simulink model "ng_pv_dynamic_dbus_p_1_sm_ng"  (Simulink 8.8)
settings: Solver=ode4  StartTime=0.0  StopTime=inf  FixedStep=0.000125  RelTol=1e-3  EnableMultiTasking=on
PreLoadFcn:
  | Ts=125e-6;Core_Num = 0; np=1; nq=1; Vmin=.9;
PostLoadFcn:
  | Ts=125e-6;Core_Num = 0; np=1; nq=1; Vmin=.9;
InitFcn:
  | Ts=125e-6;Core_Num = 0; np=1; nq=1; Vmin=.9;
undefined symbols (not defined in the file or in its folder): another_event_name, DiscIntNeverNeededParam, I, j, Left, my_event_name, Right, type, V, X
libraries: powerlib x316, simulink_extras x78, powerlib_meascontrol x47, ssn_lib x9, opal_lib x5, powerlib_extras x3, simulink x3, artemis x1, rtio_opalrt_ml605ex1 x1, rtlab x1, rtio_spectracom x1
(part 1 of 11)
settings Model: ARTEMISmethode_block_infos=$$__separator__$$ng_pv_dynamic_dbus_p_1_sm_ng/ARTEMIS Guide1$$__separator__$$  Creator=DETLDAQ  LastModifiedBy=DETLDAQ
settings OptimizationCC: BlockReduction=off  BooleanDataType=off  OptimizeBlockIOStorage=off  BufferReuse=off  GlobalBufferReuse=off  ExpressionFolding=off  LocalBlockOutputs=off
settings DebuggingCC: SaveWithParameterizedLinksMsg=none  SignalResolutionControl=TryResolveAllWithWarning  MultiTaskDSMMsg=warning  MultiTaskCondExecSysMsg=none  FcnCallInpInsideContextMsg=error
settings HardwareCC: TargetBitPerPointer=64  TargetBitPerSizeT=64  TargetBitPerPtrDiffT=64  TargetLongLongMode=on  TargetIntDivRoundTo=Zero  TargetEndianess=LittleEndian  TargetWordSize=64  TargetHWDeviceType=MATLAB Host  ProdEqTarget=off
settings RTWCC: GenCodeOnly=on
settings GRTTargetCC: CombineOutputUpdateFcns=on  GRTInterface=off

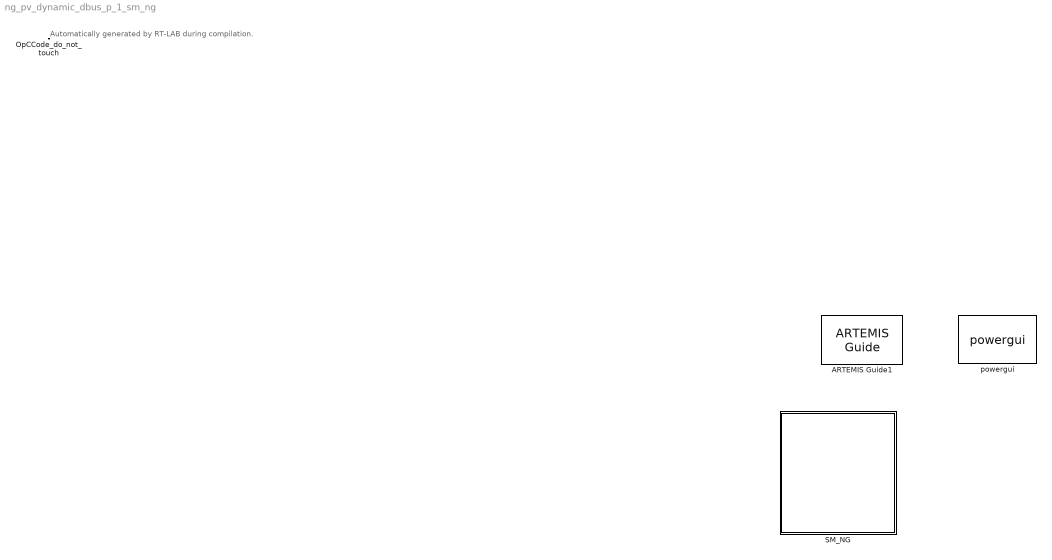
== system ng_pv_dynamic_dbus_p_1_sm_ng ==
  note: Automatically generated by RT-LAB during compilation.
  ARTEMIS Guide1 : artemis/ARTEMIS/ARTEMIS Guide  Tag=FTSSmethode_opal_4hx0r99  Description=5.0_z1  lock=on  Ts=Ts  opt=art5  dyna=off  nb_perm=4  RT_fullcomp=off  ssn=on  ssn_itvc=off  ssn_ivic=off  ssn_ext=off  ssn_solver=Backward Euler  ssn_impulse=off  ssn_quasimpulse=off  ssn_impulse_loop=5  paraExtinctionThy=off  Thy_Impulse=off  dtc=Off  dtc_opt=normal  ao=on  simtype=off  ct_mac=off  lin_mov=off  lsp=[0.001 2]  spike_skip=Disabled  dtc_extra=1  dtc_sws=normal  dtc_pied=0.5  SPSRulesBlock=SPSRules  tre=off  ctmm=off  LF=on  dpl_type=ARTEMiS DPL  rlc_type=off  custom_type=off  para=on  ssn_ImpulseLoopBlockedStateUpdate=5  ssn_mov_iter_number=5  ssn_switch_iter_number=5  ssn_nib_type_verify=on  ssn_use_lu=on  ssn_use_ldlt=off
  OpCCode_do_not_touch : opal_lib/Communication/OpCCode  SystemSampleTime=-1
  SM_NG : Subsystem
  powergui : powerlib/powergui  SimulationMode=Discrete  SolverType=Backward Euler  SampleTime=0.000125  frequency=60  SPID=off  DisableSnubberDevices=off  DisableRonSwitches=off  DisableVfSwitches=off  SwTol=0  DisplayEquations=off  Interpol=off  ExternalGateDelay=off  methode=off  Ts=100  FunctionMessages=off  echomessages=off  HookPort=off  EnableUseOfTLC=off  x0status=blocks  frequencyindice=0  Pbase=100e6  ErrMax=1e-4  Iterations=50  UnitsV=kV  UnitsW=MW  buscounter=0  RestoreLinks=warning  ResistiveCurrentMeasurement=off  Frange=[0:2:500]  Ylog=off  Xlog=on  ShowGrid=off  save=off  variable=ZData  structure=0  ZoomFFT=off  StartTime=0.0  cycles=1  DisplayStyle=1  fundamental=60  FreqAxis=off  MaxFrequency=1000  frequencyindicesteady=1  RmsSteady=1  display=off
